simulink model "heat_model"  (R2017b)
settings: Solver=VariableStepAuto  StartTime=0.0  StopTime=10.0  RelTol=1e-3
settings Model: Creator=jim  LastModifiedBy=jim

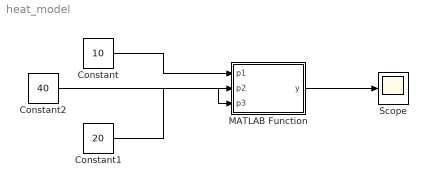
== system heat_model ==
  Constant : Constant  Value=10
  Constant1 : Constant  Value=20
  Constant2 : Constant  Value=40
  MATLAB Function : MATLAB Function  TreatAsAtomicUnit=on
  Scope : Scope
  wires:
  Constant/1 -> MATLAB Function/1(p1)
  Constant1/1 -> MATLAB Function/2(p2)
  Constant2/1 -> MATLAB Function/3(p3)
  MATLAB Function/1(y) -> Scope/1

== matlab function heat_model/MATLAB Function ==
  data: p1 input; p2 input; p3 input; y output
function y = fcn(p1, p2, p3)

y = p1 + p2 + p3;
end
